simulink model "WTE_TestBench"  (R2023b)
settings: Solver=VariableStepAuto  StartTime=0.0  StopTime=20  FixedStep=1/10000  RelTol=1e-3
undefined symbols (not defined in the file): A_c, A_d, alpha_cu, B_c, B_d, Continuous, Discrete, R_25, R_c, R_d, R_th, tau_th, Time, Ts
libraries: fl_lib x7, nesl_utility x4, simulink x3, ctrlSharedLib x2
settings Model: Creator=leoni  LastModifiedBy=leoni

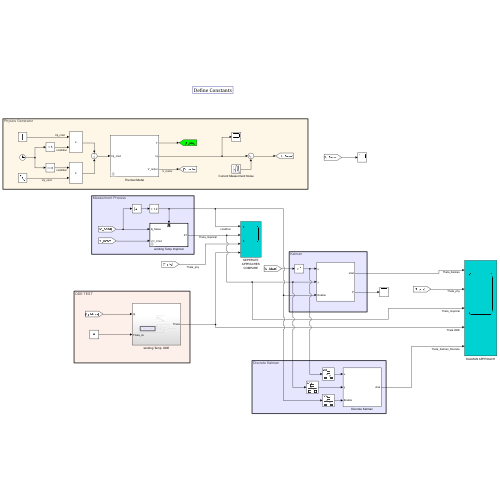
[thumbnail: Simulink's stored preview of the top-level diagram]
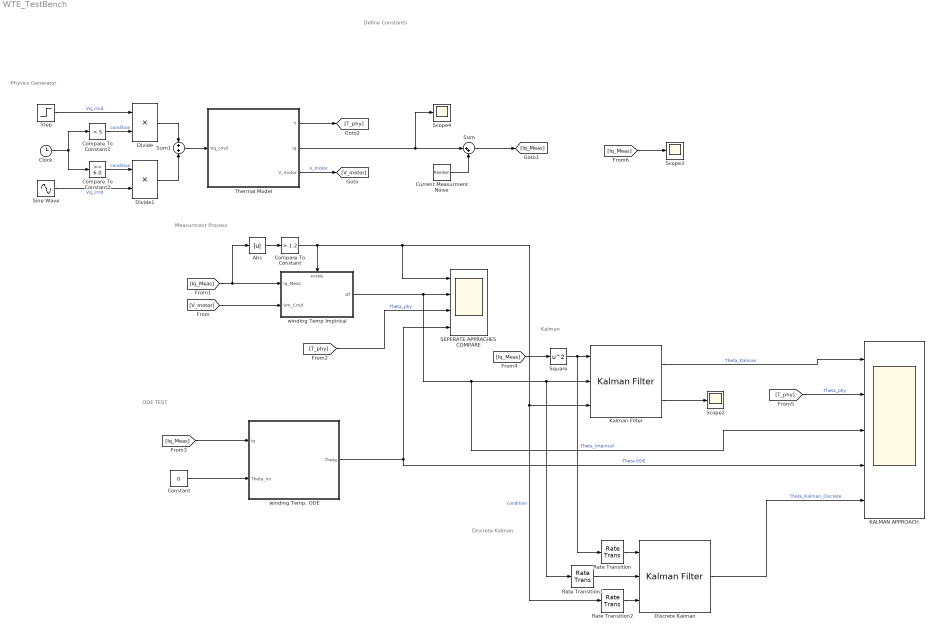
== system WTE_TestBench ==
  note: Discrete Kalman
  note: ODE TEST
  note: Kalman
  note: Measurment Process
  note: Physics Generator
  note: Define Constants
  Abs : Abs  SaturateOnIntegerOverflow=off
  Clock : Clock
  Compare To Constant : simulink/Logic and Bit Operations/Compare To Constant  relop=>  const=1.2  OutDataTypeStr=boolean
  Compare To Constant1 : simulink/Logic and Bit Operations/Compare To Constant  relop=<  const=5  OutDataTypeStr=boolean
  Compare To Constant2 : simulink/Logic and Bit Operations/Compare To Constant  relop=>=  const=6.0  OutDataTypeStr=boolean
  Constant : Constant  Value=0
  Current Measurment Noise : RandomNumber  Variance=0.1^2  SampleTime=0.001
  Discrete Kalman : ctrlSharedLib/Kalman Filter  TimeDomain=Discrete-Time  UseCurrentEstimator=on  ModelSource=Individual A, B, C, D matrices  ModelSourceVariable=ss(0.95,1,1,0,1)  A=A_d  B=B_d  C=1  D=0  NumberOfStates=1  NumberOfInputs=1  NumberOfOutputs=1  InitialEstimateSource=Dialog  X0=0  P0=10  UseK=off  UseGH=off  NumberOfProcessNoiseInputs=1  G=1  TimeInvariantG=on  H=0  TimeInvariantH=on  Q=Q_d  TimeInvariantQ=on  R=R_d  TimeInvariantR=on  N=0  TimeInvariantN=on  AddInputPort=on  AddEnablePort=on  OutputEstimatedY=off  OutputP=off  Ts=Ts
  Divide : Product  Inputs=**
  Divide1 : Product  Inputs=**
  KALMAN APPROACH : Scope  NumInputPorts=5
  Kalman Filter : ctrlSharedLib/Kalman Filter  TimeDomain=Continuous-Time  UseCurrentEstimator=on  ModelSource=Individual A, B, C, D matrices  ModelSourceVariable=ss(0.95,1,1,0,1)  A=A_c  B=B_c  C=1  D=0  NumberOfStates=1  NumberOfInputs=1  NumberOfOutputs=1  InitialEstimateSource=Dialog  X0=0  P0=10  UseK=off  UseGH=off  NumberOfProcessNoiseInputs=1  G=1  TimeInvariantG=on  H=0  TimeInvariantH=on  Q=Q_c  TimeInvariantQ=on  R=R_c  TimeInvariantR=on  N=0  TimeInvariantN=on  AddInputPort=on  AddEnablePort=on  OutputEstimatedY=off  OutputP=on  Ts=-1
  Rate Transition : RateTransition
  Rate Transition1 : RateTransition
  Rate Transition2 : RateTransition
  SEPERATE APPRACHES COMPARE : Scope  NumInputPorts=4
  Scope2 : Scope
  Scope3 : Scope
  Scope4 : Scope
  Sine Wave : Sin  Amplitude=0.6  Frequency=2*pi*2  SampleTime=0
  Square : Math  Operator=square
  Step : Step  After=0.8  SampleTime=0
  Sum : Sum  Inputs=|++
  Sum1 : Sum  Inputs=+|+
  Thermal Model : Subsystem  mask{V_bus=28}
      mask prompts: V_bus "Bus Voltage[V]"
  winding Temp Impirical : Subsystem  TreatAsAtomicUnit=on  mask{alpha_cu=alpha_cu}
      mask prompts: alpha_cu "alpha Cu [1/K]"
  winding Temp. ODE : Subsystem
  wires:
  Step/1 -> Divide/1  "Vq_cmd"
  Thermal Model/3(V_motor) -> [V_motor]  "V_motor"
  Thermal Model/2(Iq) -> Scope4/1, Sum/1
  Thermal Model/1(T) -> [T_phy]
  [V_motor] -> winding Temp Impirical/2(Vm_Cmd)
  [Iq_Meas] -> winding Temp Impirical/1(Iq_Meas), Abs/1
  Abs/1 -> Compare To Constant/1
  Compare To Constant/1 -> Kalman Filter/3, Rate Transition2/1, SEPERATE APPRACHES COMPARE/1, winding Temp Impirical/Enable  "condition"
  winding Temp Impirical/1(dT) -> KALMAN APPROACH/3, Kalman Filter/2, Rate Transition1/1, SEPERATE APPRACHES COMPARE/2  "Theta_Impirical"
  [T_phy] -> SEPERATE APPRACHES COMPARE/3  "Theta_phy"
  [Iq_Meas] -> winding Temp. ODE/1(Iq)
  Constant/1 -> winding Temp. ODE/2(Theta_ini)
  winding Temp. ODE/1(Theta) -> SEPERATE APPRACHES COMPARE/4, KALMAN APPROACH/4  "Theta ODE"
  [Iq_Meas] -> Square/1
  Kalman Filter/1 -> KALMAN APPROACH/1  "Theta_Kalman"
  [T_phy] -> KALMAN APPROACH/2  "Theta_phy"
  Kalman Filter/2 -> Scope2/1
  Sine Wave/1 -> Divide1/2  "Vq_cmd"
  Current Measurment Noise/1 -> Sum/2
  Sum/1 -> [Iq_Meas]
  [Iq_Meas] -> Scope3/1
  Clock/1 -> Compare To Constant2/1, Compare To Constant1/1
  Compare To Constant1/1 -> Divide/2  "condition"
  Compare To Constant2/1 -> Divide1/1  "condition"
  Divide1/1 -> Sum1/2
  Divide/1 -> Sum1/1
  Sum1/1 -> Thermal Model/1(Vq_cmd)
  Square/1 -> Rate Transition/1, Kalman Filter/1
  Discrete Kalman/1 -> KALMAN APPROACH/5  "Theta_Kalman_Discrete"
  Rate Transition/1 -> Discrete Kalman/1
  Rate Transition1/1 -> Discrete Kalman/2
  Rate Transition2/1 -> Discrete Kalman/3

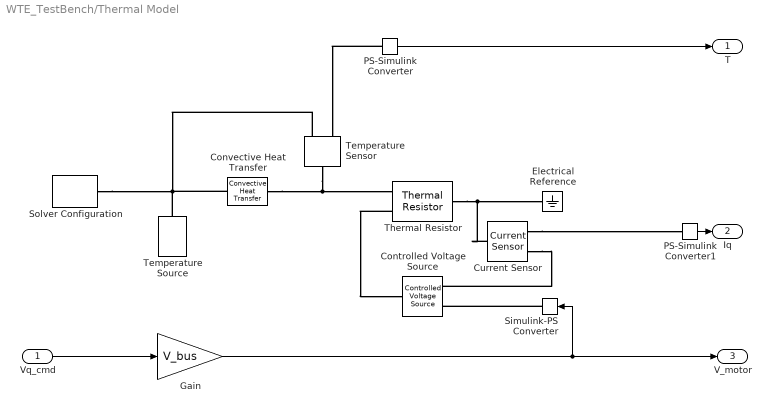
== system WTE_TestBench/Thermal Model ==
  Vq_cmd : Inport
  Controlled Voltage Source : fl_lib/Electrical/Electrical Sources/Controlled Voltage Source
  Convective Heat Transfer : fl_lib/Thermal/Thermal Elements/Convective Heat Transfer  thermal_type=foundation.enum.constant_variable.constant  area=1 m^2  heat_tr_coeff=1/25 W/(K*m^2)  min_heat_tr_coeff=1e-3 W/(K*m^2)  T_specify=off  T_priority=High  T=0 degC  T_nominal_specify=off  T_nominal_unit=K  T_nominal_value=1  Q_specify=off  Q_priority=None  Q=0 W  Q_nominal_specify=off  Q_nominal_unit=W  Q_nominal_value=1
  Current Sensor : fl_lib/Electrical/Electrical Sensors/Current Sensor
  Electrical Reference : fl_lib/Electrical/Electrical Elements/Electrical Reference
  Gain : Gain  Gain=V_bus
  PS-Simulink Converter : nesl_utility/PS-Simulink Converter  PhysicalDomain=network_engine_domain  SubClassName=ps_output  LeftPortType=input  RightPortType=output  PseudoPeriodic=off  Frequencies=[]  VectorFormat=inherit  Unit=K  AffineConversion=on
  PS-Simulink Converter1 : nesl_utility/PS-Simulink Converter  PhysicalDomain=network_engine_domain  SubClassName=ps_output  LeftPortType=input  RightPortType=output  PseudoPeriodic=off  Frequencies=[]  VectorFormat=inherit  Unit=inherit  AffineConversion=off
  Simulink-PS Converter : nesl_utility/Simulink-PS Converter  PhysicalDomain=network_engine_domain  SubClassName=ps_input  LeftPortType=input  RightPortType=output  PseudoPeriodic=off  Frequencies=[]  NoiseDistribution=none  NoiseParameters=[]  Unit=V  AffineConversion=off  FilteringAndDerivatives=provide  SimscapeFilterOrder=1  InputFilterTimeConstant=0.001  UdotUserProvided=0
  Solver Configuration : nesl_utility/Solver Configuration  PhysicalDomain=network_engine_domain  SubClassName=solver  LeftPortType=input  RightPortType=generic  Tones=[]  Harmonics=[]  SimulateNoise=off  Profile=off  UseLocalSampling=off  EnableSwitchedLinearOptims=on  FrequencyDomain=off  UseCCode=off  RelTol=0.001  AbsTol=1e-06  MinStep=1e-09  ToWorkspace=off  RevertToSquareIcSolve=off  NumHomotopyIterations=100  PhasorMode=off  PhasorModeNumHarmonics=1  ConsistencySolver=NEWTON_XTOL_AFTER_FTOL  IndexReductionMethod=DerivativeReplacement  DoDC=off  ResidualTolerance=1e-09  ConsistencyTolSource=GLOBAL  ConsistencyAbsTol=0.001  ConsistencyRelTol=0.001  ConsistencyTolFactor=0.001  UseLocalSolver=off  LocalSolverChoice=NE_TRAPEZOIDAL_ADVANCER  ResolveIndetEquations=on  FunctionEvalNumThread=1  LocalSolverSampleTime=0.001  DoFixedCost=off  MaxNonlinIter=3  MaxModeIter=2  ComputeImpulses=off  ImpulseIterations=2  LinearAlgebra=auto  LinearAlgebraNumThread=0  EquationFormulation=NE_TIME_EF  DelaysMemoryBudget=1024  AutomaticFiltering=on  FilteringTimeConstant=0.001  PartitionStorageMethod=AS_NEEDED  PartitionMemoryBudget=1024  PartitionMethod=ROBUST  MultibodyUseLocalSolver=off  MultibodyLocalSolverChoice=ODE1  MultibodyLocalSolverSampleTime=0.001
  Temperature Sensor : fl_lib/Thermal/Thermal Sensors/Temperature Sensor  temperature_measure=foundation.enum.MeasurementReference.difference
  Temperature Source : fl_lib/Thermal/Thermal Sources/Temperature Source  temperature=25 degC
  Thermal Resistor : fl_lib/Electrical/Electrical Elements/Thermal Resistor  R0=7.0 Ohm  T0=25 degC  alpha=alpha_cu 1/K  tc=tau_th s  K_d=1/R_th W/K  T_specify=on  T_priority=High  T=50 degC  T_nominal_specify=off  T_nominal_unit=K  T_nominal_value=1
      settings: InternalSimscapePortConfiguration="{\"Bottom\":[],\"Left\":[{\"id\":\"H\",\"label\":\"H\",\"type\":\"foundation.thermal.thermal\"},{\"id\":\"p\",\"label\":\"+\",\"type\":\"foundation.electrical.electrical\"}],\"Right\":[{\"id\":\"n\",\"label\":\"-\",\"type\":\"foundation.electrical.electrical\"}],\"Top\":[]}"
  T : Outport
  Iq : Outport  Port=2
  V_motor : Outport  Port=3
  wires:
  Vq_cmd/1 -> Gain/1
  PS-Simulink Converter/1 -> T/1
  PS-Simulink Converter1/1 -> Iq/1
  Gain/1 -> V_motor/1, Simulink-PS Converter/1
  connections:
  Thermal Resistor/LConn2 -- Controlled Voltage Source/LConn1
  Solver Configuration/RConn1 -- Convective Heat Transfer/RConn1 -- Temperature Sensor/RConn1 -- Temperature Source/LConn1
  Convective Heat Transfer/LConn1 -- Temperature Sensor/LConn1 -- Thermal Resistor/LConn1
  Simulink-PS Converter/RConn1 -- Controlled Voltage Source/RConn1
  Thermal Resistor/RConn1 -- Current Sensor/LConn1 -- Electrical Reference/LConn1
  Current Sensor/RConn1 -- PS-Simulink Converter1/LConn1
  Current Sensor/RConn2 -- Controlled Voltage Source/RConn2
  PS-Simulink Converter/LConn1 -- Temperature Sensor/RConn2

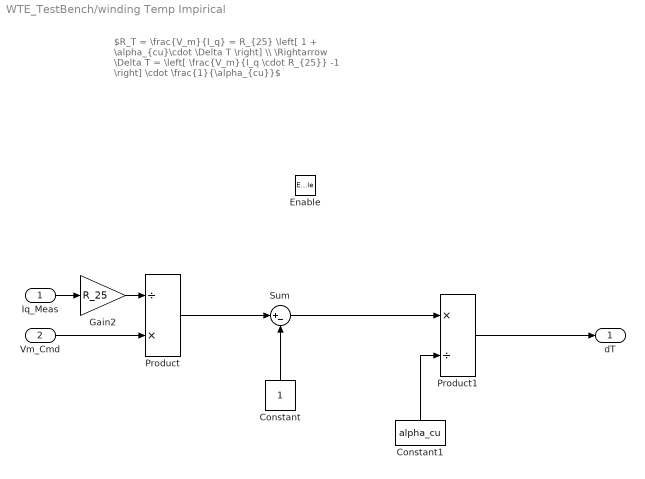
== system WTE_TestBench/winding Temp Impirical ==
  note: $R_T = \frac{V_m}{I_q} = R_{25} \left[ 1 + \alpha_{cu}\cdot \Delta T \right] \\ \Rightarrow \Delta T = \left[ \frac{V_m}{I_q \cdot R_{25}} -1 \right] \cdot \frac{1}{\alpha_{cu}}$
  Iq_Meas : Inport
  Vm_Cmd : Inport  Port=2
  Enable : EnablePort
  Constant : Constant
  Constant1 : Constant  Value=alpha_cu
  Gain2 : Gain  Gain=R_25
  Product : Product  Inputs=/*
  Product1 : Product  Inputs=*/
  Sum : Sum  Inputs=|+-
  dT : Outport
  wires:
  Iq_Meas/1 -> Gain2/1
  Vm_Cmd/1 -> Product/2
  Product/1 -> Sum/1
  Constant/1 -> Sum/2
  Sum/1 -> Product1/1
  Constant1/1 -> Product1/2
  Product1/1 -> dT/1
  Gain2/1 -> Product/1

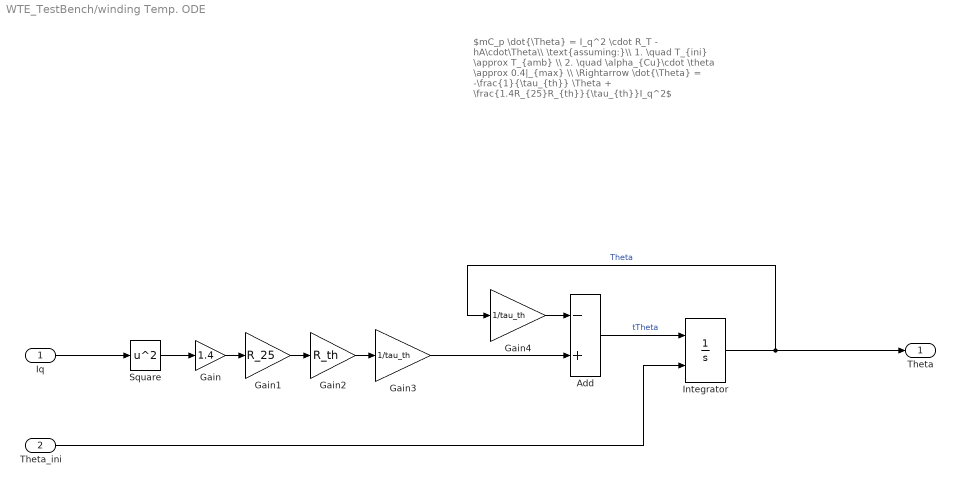
== system WTE_TestBench/winding Temp. ODE ==
  note: $mC_p \dot{\Theta} = I_q^2 \cdot R_T - hA\cdot\Theta\\ \text{assuming:}\\ 1. \quad T_{ini} \approx T_{amb} \\ 2. \quad \alpha_{Cu}\cdot \theta \approx 0.4|_{max} \\ \Rightarrow \dot{\Theta} = -\frac{1}{\tau_{th}} \Theta + \frac{1.4R_{25}R_{th}}{\tau_{th}}I_q^2$
  Iq : Inport
  Theta_ini : Inport  Port=2
  Add : Sum  Inputs=-+
  Gain : Gain  Gain=1.4
  Gain1 : Gain  Gain=R_25
  Gain2 : Gain  Gain=R_th
  Gain3 : Gain  Gain=1/tau_th
  Gain4 : Gain  Gain=1/tau_th
  Integrator : Integrator  InitialConditionSource=external
  Square : Math  Operator=square
  Theta : Outport
  wires:
  Iq/1 -> Square/1
  Integrator/1 -> Gain4/1, Theta/1  "Theta"
  Add/1 -> Integrator/1  "tTheta"
  Gain/1 -> Gain1/1
  Gain1/1 -> Gain2/1
  Gain2/1 -> Gain3/1
  Square/1 -> Gain/1
  Gain3/1 -> Add/2
  Gain4/1 -> Add/1
  Theta_ini/1 -> Integrator/2
